simulink model "G3P3_Demo"  (R2019b)
settings: Solver=VariableStepAuto  StartTime=0.0  StopTime=3600*24  RelTol=1e-3
undefined symbols (not defined in the file or in its folder): sigbuilder_block
libraries: powerlib x1
settings Model: Creator=Owner  LastModifiedBy=Owner

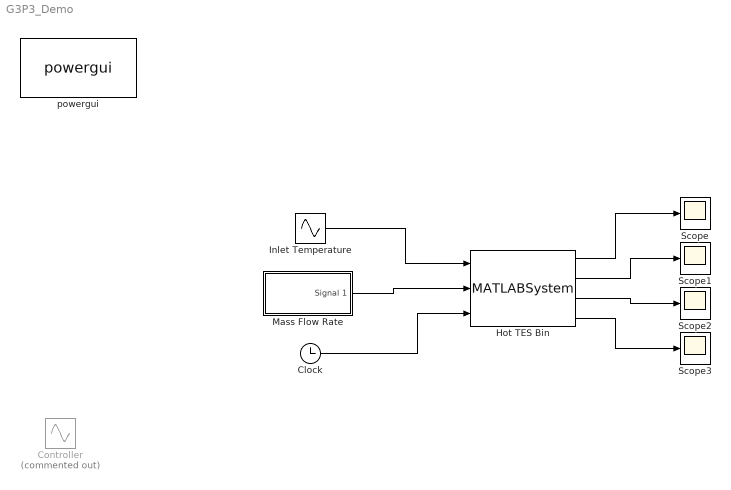
== system G3P3_Demo ==
  Clock : Clock
  Controller : Sin  Commented=on  Amplitude=200  Bias=400  Frequency=0.0001  Phase=pi  SampleTime=0
  Hot TES Bin : MATLABSystem  System=TES  SimulateUsing=Interpreted execution  Hp=7  bp=0.3214  a=0.01  h=0.025  T0=800  Tinf=20  Tref=0  hInf=10  hcw=1  hcwA=1  tauW1=1.7057e-04  hp1=10  hp2=10  hp3=10  hp4=10  hp5=10  hp5D=2  hp5H=2  hp5C=2  hpTop=5  kp=0.4  rhopPack=2000  rhopLoose=1810  cpp=1025.965  mup=2.5 * 1.81e-5
      mask Type: TES
      mask Display:
      | disp('TES');
      | port_label('input',1,'Tin');
      | port_label('input',2,'mdot');
      | port_label('input',3,'t');
      | port_label('output',1,'Tout');
      | port_label('output',2,'Tbulk');
      | port_label('output',3,'Estored');
      | port_label('output',4,'ztop');
  Inlet Temperature : Sin  Amplitude=20  Bias=700  Frequency=0.0001  SampleTime=0
  Mass Flow Rate : Subsystem  Tag=STV Subsys  LoadFcn=sigbuilder_block('load');  StartFcn=sigbuilder_block('start');  StopFcn=sigbuilder_block('stop');  ClipboardFcn=sigbuilder_block('clipboard');  mask(Sigbuilder block){tuvar=[0:10]}
      mask help: Simulink:masks:SigbuilderBlock_MD
      mask init:
      | if ~strcmp(get_param(bdroot(gcbh),'SimulationStatus'),'stopped') tuvar = sigbuilder_block('maskInit'); end
      settings: CopyFcn=sigbuilder_block('copy');  DeleteFcn=sigbuilder_block('delete');  ModelCloseFcn=sigbuilder_block('modelClose');  PreSaveFcn=sigbuilder_block('preSave');  PauseFcn=sigbuilder_block('pause');  ContinueFcn=sigbuilder_block('continue');  NameChangeFcn=sigbuilder_block('namechange');  OpenFcn=sigbuilder_block('open',[437.6 199.2 550.4 400 ]);  CloseFcn=sigbuilder_block('close');
      mask Display: plot(0, 0, 100, 100,[2, 2, 32, 32, 2], [68, 8, 8, 68, 68],[32, 2], [38, 38], [32, 19, 2],[53, 60, 44], [32, 17, 17, 2],[16, 16, 31, 31]);txt = getActiveGroup(gcbh);text(2, 100, txt,'verticalAlignment', 'top');
  Scope{,1..3} (4 alike) : Scope
  powergui : powerlib/powergui  Priority=1  SimulationMode=Discrete  SampleTime=1  frequency=60  Iterations=50  frequencyindice=0  Pbase=100e6  ErrMax=1e-4  UnitsV=kV  UnitsW=MW  buscounter=0  FunctionMessages=off  echomessages=off  EnableUseOfTLC=off  CurrentSourceSwitches=off  DisableSnubberDevices=off  DisableRonSwitches=off  DisableVfSwitches=off  DisplayEquations=off  AutomaticDiscreteSolvers=off  SolverType=Tustin/Backward Euler (TBE)  Interpol=off  ExternalGateDelay=off  methode=off  Ts=100  x0status=blocks  SPID=on  SwTol=0  HookPort=off  NonlinearTolerance=1e-4  nMaxIteration=100  ContinueOnMaxIteration=off  RestoreLinks=warning  ResistiveCurrentMeasurement=off  Frange=[0:2:500]  Ylog=off  Xlog=on  ShowGrid=off  save=off  variable=ZData  structure=0  ZoomFFT=off  StartTime=0.0  cycles=1  DisplayStyle=1  fundamental=60  FreqAxis=off  MaxFrequency=1000  frequencyindicesteady=1  RmsSteady=1  display=off
      settings: SourceProductName=Simscape Electrical
  wires:
  Inlet Temperature/1 -> Hot TES Bin/1
  Hot TES Bin/1 -> Scope/1
  Clock/1 -> Hot TES Bin/3
  Mass Flow Rate/1(Signal 1) -> Hot TES Bin/2
  Hot TES Bin/2 -> Scope1/1
  Hot TES Bin/3 -> Scope2/1
  Hot TES Bin/4 -> Scope3/1

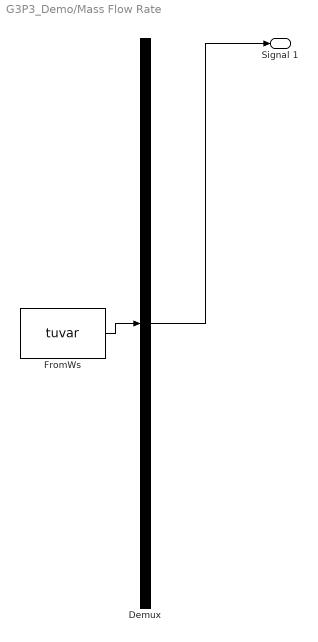
== system G3P3_Demo/Mass Flow Rate ==
  Demux : Demux  Tag=STV Demux  Outputs=1
  FromWs : FromWorkspace  Tag=STV FromWs  VariableName=tuvar  SampleTime=0
      SigBuilderData=|
      | common.afterFinalStr = 'Extrapolate'
      | common.sampleTime = 0
      | dataSet.timeRange = [0 24]
      | dataSet.name = 'Group 1'
      | sbobj.Groups.Name = 'Group 1'
      | sbobj.Groups.Signals.Name = 'Signal 1'
      | sbobj.Groups.Signals.XData = [0 6 6 16 16 24]
      | sbobj.Groups.Signals.YData = [9 9 0 0 -5 -5]
      | sbobj.Groups.TimeRange = [0 24]
  Signal 1 : Outport  Tag=STV Outport
  wires:
  Demux/1 -> Signal 1/1
  FromWs/1 -> Demux/1
